simulink model "wimax_system_simulation"  (Simulink 6.1)
settings: Solver=ode45  StartTime=0.0  StopTime=inf  FixedStep=Auto  RelTol=1e-3
libraries: simulink x8, dspsrcs4 x6, dspindex x4, dspbuff3 x4, commchan2 x2, commutil2 x2, dspxfrm3 x2, dspmtrx3 x2, commcnvcod2 x2, commblkintrlv2 x2, commdigbbndam2 x2, commrandsrc2 x1
settings Model: LastModifiedBy=shaikh.m
settings DebuggingCC: SolverPrmCheckMsg=warning

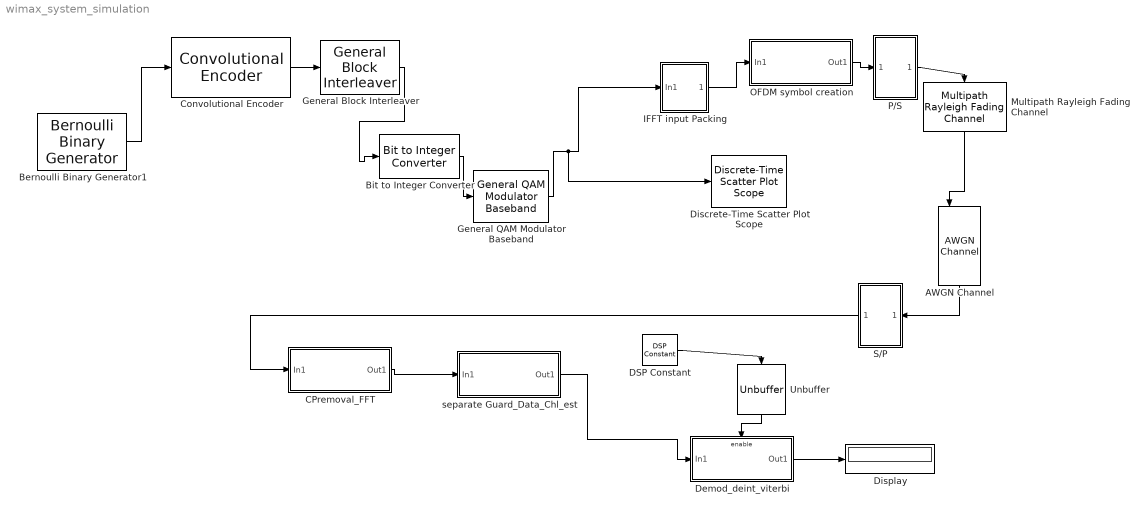
== system wimax_system_simulation ==
  AWGN Channel : commchan2/AWGN Channel  Orientation=down  seed=67  noiseMode=Variance from port  EbNodB=10  EsNodB=10  SNRdB=30  bitsPerSym=1  Ps=1  Tsym=1  variance=1
  Bernoulli Binary Generator1 : commrandsrc2/Bernoulli Binary Generator  P=0.5  seed=93  Ts=0.05e-6  frameBased=on  sampPerFrame=384  orient=off
      link override Random Source: MinVal=zeros(size(P))  MaxVal=ones(size(P))  SampTime=0.05e-6
  Bit to Integer Converter : commutil2/Bit to Integer Converter  nbits=4
  CPremoval_FFT : Subsystem
  Convolutional Encoder : commcnvcod2/Convolutional Encoder  trellis=poly2trellis(7, [171 133])  reset=On each frame
  DSP Constant : dspsrcs4/DSP Constant  Value=1  SampleMode=Discrete  discreteOutput=Sample-based  continuousOutput=Sample-based  sampTime=0.05e-6  framePeriod=2  dataType=Inherit from 'Constant value'  isSigned=on  wordLen=16  udDataType=sfix(16)  fracBitsMode=Best precision  numFracBits=15  InterpretAs1D=-inf  Ts=-inf  FramebasedOutput=-inf
  Demod_deint_viterbi : Subsystem  TreatAsAtomicUnit=on
  Discrete-Time Scatter Plot Scope : commsink2/Discrete-Time Scatter Plot Scope  Tag=ScatterPlot  sampPerSymb=1  offsetEye=0  numTraces=40  numNewFrames=10  LineMarkers=.  LineColors=[1 0 0]  fading=on  render=on  AxisGrid=on  xMin=-1.04355162785557  xMax=1.04829504434582  yMin=-1.04592333610069  yMax=1.04592333610069  inphaseLabel=In-phase Amplitude  quadratureLabel=Quadrature Amplitude  openScopeAtSimStart=on  FrameNumber=off  FigPos=[232 106 560 560]  figTitle=Scatter Plot  numLinesMax=8  block_type_=scatter
  Display : Display
  General Block Interleaver : commblkintrlv2/General Block Interleaver  elements=jk.'
  General QAM Modulator Baseband : commdigbbndam2/General QAM Modulator Baseband  SigCon=qamConst  numSamp=1
  IFFT input Packing : Subsystem
  Multipath Rayleigh Fading Channel : commchan2/Multipath Rayleigh Fading Channel  Orientation=down  Fd=14  simTs=0.025e-6  delayVec=[0 200e-9 800e-9 1200e-9 2300e-9 3700e-9]  gainVecdB=[0 -0.9 -4.9 -8.0 -7.8 -23.9 ]  normGain=on  Seed=936497248
  OFDM symbol creation : Subsystem
  P/S : Subsystem
      mask Display: disp('P/S');
  S/P : Subsystem  Orientation=left
      mask Display: disp('S/P')
  Unbuffer : dspbuff3/Unbuffer  Orientation=down  ic=0
  separate Guard_Data_Chl_est : Subsystem
  wires:
  Convolutional Encoder/1 -> General Block Interleaver/1
  IFFT input Packing/1(Out1) -> OFDM symbol creation/1(In1)
  CPremoval_FFT/1(Out1) -> separate Guard_Data_Chl_est/1(In1)
  General QAM Modulator Baseband/1 -> IFFT input Packing/1(In1), Discrete-Time Scatter Plot Scope/1
  General Block Interleaver/1 -> Bit to Integer Converter/1
  Bit to Integer Converter/1 -> General QAM Modulator Baseband/1
  separate Guard_Data_Chl_est/1(Out1) -> Demod_deint_viterbi/1(In1)
  DSP Constant/1 -> Unbuffer/1
  Unbuffer/1 -> Demod_deint_viterbi/Enable
  AWGN Channel/1 -> S/P/1(In1)
  OFDM symbol creation/1(Out1) -> P/S/1(In1)
  Multipath Rayleigh Fading Channel/1 -> AWGN Channel/1
  P/S/1(Out1) -> Multipath Rayleigh Fading Channel/1
  S/P/1(Out1) -> CPremoval_FFT/1(In1)
  Bernoulli Binary Generator1/1 -> Convolutional Encoder/1
  Demod_deint_viterbi/1(Out1) -> Display/1

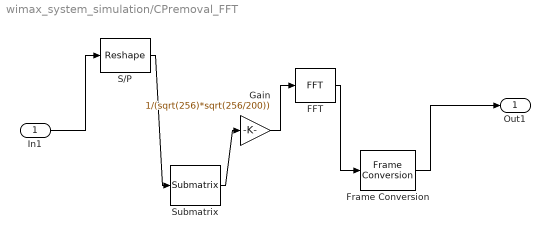
== system wimax_system_simulation/CPremoval_FFT ==
  In1 : Inport  Port=1  LatchInput=off
  FFT : dspxfrm3/FFT  DialogController=dspDDGCreate  DialogControllerArgs=DataTag0  CompMethod=Table lookup  TableOpt=Speed  BitRevOrder=off  SkipNorm=on  roundingMode=Floor  overflowMode=off
  Frame Conversion : FrameConversion
  Gain : Gain  Gain=1/(sqrt(256)*sqrt(256/200))
  S/P : simulink/Math Operations/Reshape  OutputDimensionality=Customize  OutputDimensions=[288,2]
  Submatrix : dspmtrx3/Submatrix  RowSpan=Range of rows  RowStartMode=First  RowStartIndex=31  RowEndMode=Index  RowEndIndex=256  ColSpan=All columns  ColStartMode=First  ColStartIndex=1  ColEndMode=Last  ColEndIndex=1
  Out1 : Outport
  wires:
  In1/1 -> S/P/1
  S/P/1 -> Submatrix/1
  Submatrix/1 -> Gain/1
  Gain/1 -> FFT/1
  FFT/1 -> Frame Conversion/1
  Frame Conversion/1 -> Out1/1

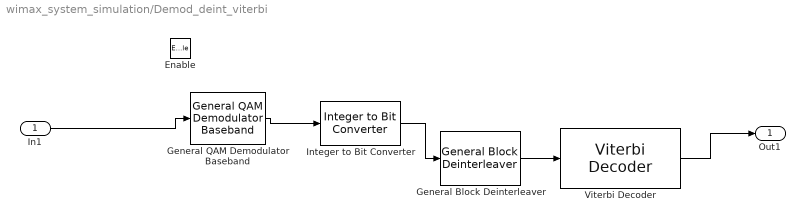
== system wimax_system_simulation/Demod_deint_viterbi ==
  In1 : Inport  Port=1  LatchInput=off
  Enable : EnablePort
  General Block Deinterleaver : commblkintrlv2/General Block Deinterleaver  elements=jk.'
  General QAM Demodulator Baseband : commdigbbndam2/General QAM Demodulator Baseband  SigCon=qamConst  numSamp=1
  Integer to Bit Converter : commutil2/Integer to Bit Converter  nbits=4
  Viterbi Decoder : commcnvcod2/Viterbi Decoder  trellis=poly2trellis(7, [171 133])  dectype=Hard Decision  nsdecb=3  tbdepth=78  opmode=Terminated  reset=off
  Out1 : Outport
  wires:
  General Block Deinterleaver/1 -> Viterbi Decoder/1
  General QAM Demodulator Baseband/1 -> Integer to Bit Converter/1
  Integer to Bit Converter/1 -> General Block Deinterleaver/1
  In1/1 -> General QAM Demodulator Baseband/1
  Viterbi Decoder/1 -> Out1/1

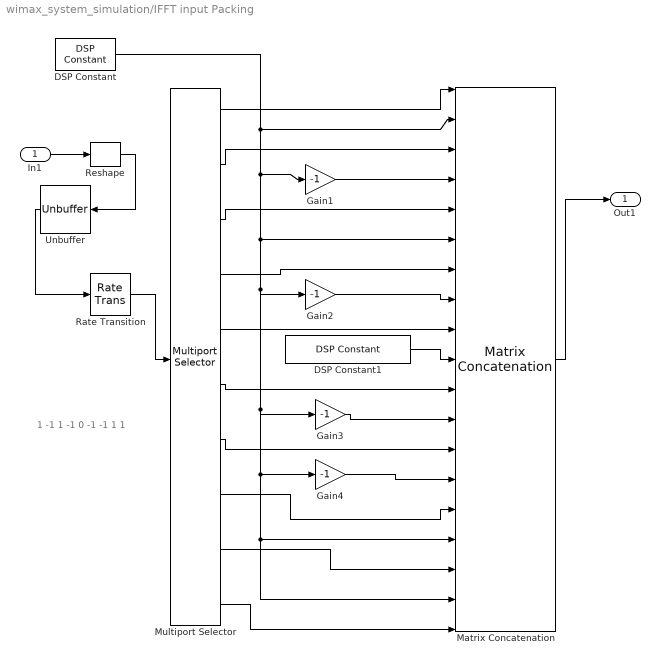
== system wimax_system_simulation/IFFT input Packing ==
  note: 1 -1 1 -1 0 -1 -1 1 1
  In1 : Inport  Port=1  LatchInput=off
  DSP Constant : dspsrcs4/DSP Constant  Value=ones(1,1)  SampleMode=Discrete  discreteOutput=Sample-based  continuousOutput=Sample-based  sampTime=0.05e-6  framePeriod=2  dataType=Inherit from 'Constant value'  isSigned=on  wordLen=16  udDataType=sfix(16)  fracBitsMode=Best precision  numFracBits=15  InterpretAs1D=-inf  Ts=-inf  FramebasedOutput=-inf
  DSP Constant1 : dspsrcs4/DSP Constant  Value=complex(0,0)*ones(1,1)  SampleMode=Discrete  discreteOutput=Sample-based  continuousOutput=Sample-based  sampTime=0.05e-6  framePeriod=2  dataType=Inherit from 'Constant value'  isSigned=on  wordLen=16  udDataType=sfix(16)  fracBitsMode=Best precision  numFracBits=15  InterpretAs1D=-inf  Ts=-inf  FramebasedOutput=-inf
  Gain{1..4} (4 alike) : Gain  Gain=-1
  Matrix Concatenation : simulink/Math Operations/Matrix Concatenation  numInports=19  catMethod=Vertical
  Multiport Selector : dspindex/Multiport Selector  rowsOrCols=Rows  idxCellArray={ 1:12, 14:37, 39:62, 64:87, 89:100, 102:113, 115:138, 140:163, 165:188, 190:201}  idxErrMode=Clip Index
  Rate Transition : RateTransition
  Reshape : simulink/Math Operations/Reshape  OutputDimensionality=Column vector  OutputDimensions=[1,1]
  Unbuffer : dspbuff3/Unbuffer  Orientation=left  ic=0
  Out1 : Outport
  wires:
  Matrix Concatenation/1 -> Out1/1
  DSP Constant/1 -> Matrix Concatenation/2, Gain1/1, Matrix Concatenation/6, Gain2/1, Gain3/1, Gain4/1, Matrix Concatenation/16, Matrix Concatenation/18
  Multiport Selector/2 -> Matrix Concatenation/3
  Gain1/1 -> Matrix Concatenation/4
  Multiport Selector/3 -> Matrix Concatenation/5
  Multiport Selector/4 -> Matrix Concatenation/7
  Gain2/1 -> Matrix Concatenation/8
  Multiport Selector/5 -> Matrix Concatenation/9
  DSP Constant1/1 -> Matrix Concatenation/10
  Multiport Selector/1 -> Matrix Concatenation/1
  Multiport Selector/6 -> Matrix Concatenation/11
  Gain3/1 -> Matrix Concatenation/12
  Multiport Selector/7 -> Matrix Concatenation/13
  Gain4/1 -> Matrix Concatenation/14
  Multiport Selector/8 -> Matrix Concatenation/15
  Multiport Selector/9 -> Matrix Concatenation/17
  Multiport Selector/10 -> Matrix Concatenation/19
  In1/1 -> Reshape/1
  Reshape/1 -> Unbuffer/1
  Rate Transition/1 -> Multiport Selector/1
  Unbuffer/1 -> Rate Transition/1

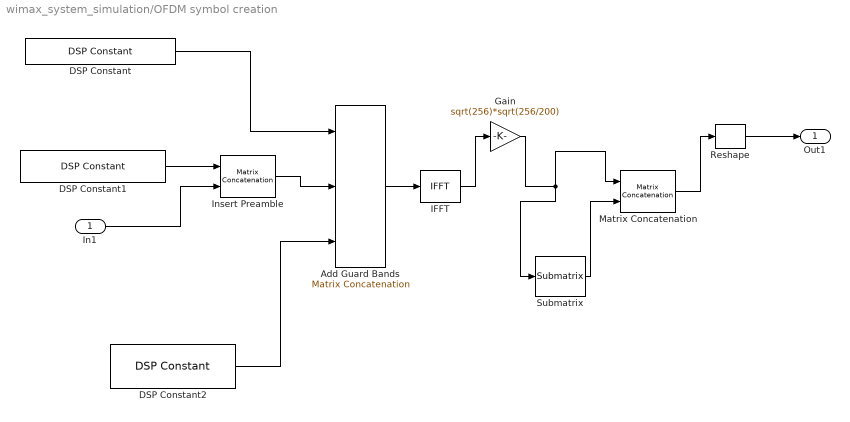
== system wimax_system_simulation/OFDM symbol creation ==
  In1 : Inport  Port=1  LatchInput=off
  Add Guard Bands : simulink/Math Operations/Matrix Concatenation  numInports=3  catMethod=Vertical
  DSP Constant : dspsrcs4/DSP Constant  Value=complex(0,0)*ones(28,2)  SampleMode=Discrete  discreteOutput=Sample-based  continuousOutput=Sample-based  sampTime=0.05e-6  framePeriod=2  dataType=Inherit from 'Constant value'  isSigned=on  wordLen=16  udDataType=sfix(16)  fracBitsMode=Best precision  numFracBits=15  InterpretAs1D=-inf  Ts=-inf  FramebasedOutput=-inf
  DSP Constant1 : dspsrcs4/DSP Constant  Value=complex(ones(201,1))  SampleMode=Discrete  discreteOutput=Sample-based  continuousOutput=Sample-based  sampTime=0.05e-6  framePeriod=2  dataType=Inherit from 'Constant value'  isSigned=on  wordLen=16  udDataType=sfix(16)  fracBitsMode=Best precision  numFracBits=15  InterpretAs1D=-inf  Ts=-inf  FramebasedOutput=-inf
  DSP Constant2 : dspsrcs4/DSP Constant  Value=complex(0,0)*ones(27,2)  SampleMode=Discrete  discreteOutput=Sample-based  continuousOutput=Sample-based  sampTime=0.05e-6  framePeriod=2  dataType=Inherit from 'Constant value'  isSigned=on  wordLen=16  udDataType=sfix(16)  fracBitsMode=Best precision  numFracBits=15  InterpretAs1D=-inf  Ts=-inf  FramebasedOutput=-inf
  Gain : Gain  Gain=sqrt(256)*sqrt(256/200)
  IFFT : dspxfrm3/IFFT  DialogController=dspDDGCreate  DialogControllerArgs=DataTag1  CompMethod=Table lookup  TableOpt=Speed  BitRevOrder=off  cs_in=off  SkipNorm=off  mode=Complex  roundingMode=Floor  overflowMode=off
  Insert Preamble : simulink/Math Operations/Matrix Concatenation  numInports=2  catMethod=Horizontal
  Matrix Concatenation : simulink/Math Operations/Matrix Concatenation  numInports=2  catMethod=Vertical
  Reshape : simulink/Math Operations/Reshape  OutputDimensionality=Column vector  OutputDimensions=[1,1]
  Submatrix : dspmtrx3/Submatrix  RowSpan=Range of rows  RowStartMode=Offset from last  RowStartIndex=31  RowEndMode=Last  RowEndIndex=1  ColSpan=All columns  ColStartMode=First  ColStartIndex=1  ColEndMode=Last  ColEndIndex=1
  Out1 : Outport
  wires:
  DSP Constant1/1 -> Insert Preamble/1
  In1/1 -> Insert Preamble/2
  DSP Constant/1 -> Add Guard Bands/1
  Insert Preamble/1 -> Add Guard Bands/2
  DSP Constant2/1 -> Add Guard Bands/3
  Add Guard Bands/1 -> IFFT/1
  IFFT/1 -> Gain/1
  Gain/1 -> Matrix Concatenation/1, Submatrix/1
  Submatrix/1 -> Matrix Concatenation/2
  Matrix Concatenation/1 -> Reshape/1
  Reshape/1 -> Out1/1

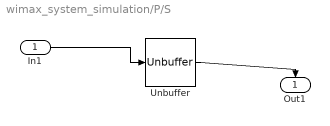
== system wimax_system_simulation/P/S ==
  In1 : Inport  Port=1  LatchInput=off
  Unbuffer : dspbuff3/Unbuffer  ic=0
  Out1 : Outport  Orientation=down
  wires:
  Unbuffer/1 -> Out1/1
  In1/1 -> Unbuffer/1

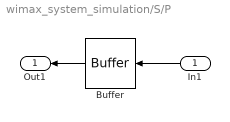
== system wimax_system_simulation/S/P ==
  In1 : Inport  Orientation=left  Port=1  LatchInput=off
  Buffer : dspbuff3/Buffer  Orientation=left  N=576  V=0  ic=0
  Out1 : Outport  Orientation=left
  wires:
  In1/1 -> Buffer/1
  Buffer/1 -> Out1/1

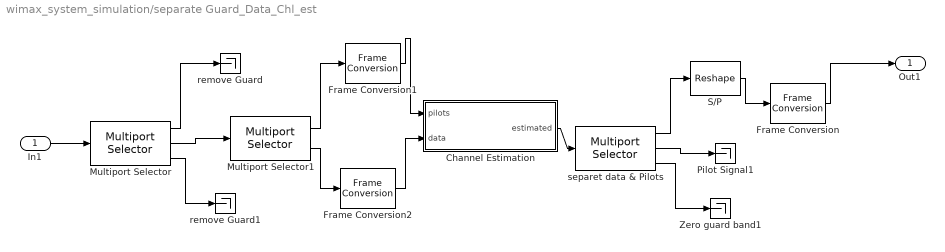
== system wimax_system_simulation/separate Guard_Data_Chl_est ==
  In1 : Inport  Port=1  LatchInput=off
  Channel Estimation : Stateflow chart
  Frame Conversion : FrameConversion
  Frame Conversion1 : FrameConversion  OutFrame=Sample based
  Frame Conversion2 : FrameConversion  OutFrame=Sample based
  Multiport Selector : dspindex/Multiport Selector  rowsOrCols=Rows  idxCellArray={ 1:28,29:229,230:256 }  idxErrMode=Clip Index
  Multiport Selector1 : dspindex/Multiport Selector  rowsOrCols=Columns  idxCellArray={1,2}  idxErrMode=Clip Index
  Pilot Signal1 : Terminator
  S/P : simulink/Math Operations/Reshape  OutputDimensionality=Column vector  OutputDimensions=[288,2]
  Zero guard band1 : Terminator
  remove Guard : Terminator
  remove Guard1 : Terminator
  separet data & Pilots : dspindex/Multiport Selector  rowsOrCols=Rows  idxCellArray={ [1:12, 14:37, 39:62, 64:87, 89:100, 102:113, 115:138, 140:163, 165:188, 190:201],[13,38,63,88,114,139,164,189],[101]}  idxErrMode=Clip Index
  Out1 : Outport
  wires:
  In1/1 -> Multiport Selector/1
  Multiport Selector/1 -> remove Guard/1
  Multiport Selector/3 -> remove Guard1/1
  Multiport Selector/2 -> Multiport Selector1/1
  Channel Estimation/1(estimated) -> separet data & Pilots/1
  separet data & Pilots/1 -> S/P/1
  separet data & Pilots/2 -> Pilot Signal1/1
  separet data & Pilots/3 -> Zero guard band1/1
  Multiport Selector1/1 -> Frame Conversion1/1
  Frame Conversion1/1 -> Channel Estimation/1(pilots)
  Multiport Selector1/2 -> Frame Conversion2/1
  Frame Conversion2/1 -> Channel Estimation/2(data)
  S/P/1 -> Frame Conversion/1
  Frame Conversion/1 -> Out1/1

== matlab function separate Guard_Data_Chl_est/Channel Estimation ==
  data: pilots input inherited; estimated output inherited; data input inherited
function estimated = fcn(pilots, data)
% This block supports the Embedded MATLAB subset.
x=complex(ones(201,1));
h_est=pilots./x;
estimated = data./h_est;
